simulink model "Couple_Tank"  (R2018b)
settings: Solver=ode5  StartTime=0.0  StopTime=1000  FixedStep=0.01  RelTol=1e-3  EnableMultiTasking=on
undefined symbols (not defined in the file or in its folder): sgn
settings Model: Creator=DUYLINH  LastModifiedBy=daiba
settings DataIOCC: LimitDataPoints=on  SaveFormat=Array
settings OptimizationCC: LifeSpan=inf
settings DebuggingCC: SFUnexpectedBacktrackingDiag=warning  SFNoUnconditionalDefaultTransitionDiag=warning  SFExecutionAtInitializationDiag=none
settings HardwareCC: ProdBitPerPointer=32  ProdBitPerSizeT=32  ProdBitPerPtrDiffT=32  ProdLargestAtomicFloat=None  ProdIntDivRoundTo=Undefined  ProdEndianess=Unspecified  ProdWordSize=32  ProdHWDeviceType=32-bit Generic
settings ModelReferenceCC: PropagateSignalLabelsOutOfModel=off
settings SFSimCC: SimUseLocalCustomCode=off
settings RTWCC: RTWUseLocalCustomCode=off
settings CodeAppCC: StateflowObjectComments=on
settings GRTTargetCC: TargetLangStandard=C89/C90 (ANSI)  GeneratePreprocessorConditionals=Disable all
settings ConfigComp: CovMetricSettings=dw  CovHtmlReporting=on  CovSaveCumulativeToWorkspaceVar=on  CovSaveSingleToWorkspaceVar=on  CovExternalEMLEnable=off

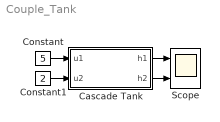
== system Couple_Tank ==
  " Cascade Tank" : Subsystem  mask{AA1=15, AA2=10, a1=0.3, a2=0.15, a12=0.1, k1=0.25, k2=0.2, Cd1=0.6, Cd2=0.6, Cd12=0.5, g=9.81, h1_zero=1, h2_zero=0.5}
      mask prompts: AA1 "Tiet dien ngang tank_1"; AA2 "Tiet dien ngang tank_2"; a1 "Tiet dien van xa tank_1"; a2 "Tiet dien van xa tank_2"; a12 "Tiet dien van xa giua 2 tank"; k1 "He so ti le cong suat may bom 1"; k2 "He so ti le cong suat may bom 2"; Cd1 "He so xa tank_1"; Cd2 "He so xa tank_2"; Cd12 "He so xa giua 2 tank"; g "Gia toc trong truong"; h1_zero "Muc nuoc tank_1 ban dau"; h2_zero "Muc nuoc tank_2 ban dau"
  Constant : Constant  Value=5
  Constant1 : Constant  Value=2
  Scope : Scope  NumInputPorts=2
  wires:
  " Cascade Tank"/1(h1) -> Scope/1
  Constant/1 -> " Cascade Tank"/1(u1)
  " Cascade Tank"/2(h2) -> Scope/2
  Constant1/1 -> " Cascade Tank"/2(u2)

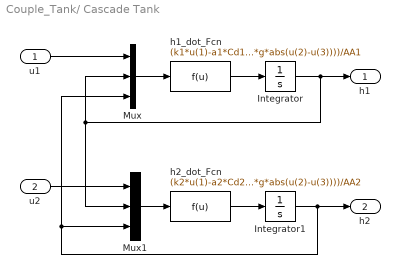
== system Couple_Tank/ Cascade Tank ==
  u1 : Inport
  u2 : Inport  Port=2
  Integrator : Integrator  InitialCondition=h1_zero
  Integrator1 : Integrator  InitialCondition=h2_zero
  Mux : Mux  Inputs=3
  Mux1 : Mux  Inputs=3
  h1_dot_Fcn : Fcn  Expr=(k1*u(1)-a1*Cd1*sqrt(2*g*u(2))-Cd12*sgn(u(2)-u(3))*a12*sqrt(2*g*abs(u(2)-u(3))))/AA1
  h2_dot_Fcn : Fcn  Expr=(k2*u(1)-a2*Cd2*sqrt(2*g*u(3))-Cd12*sgn(u(3)-u(2))*a12*sqrt(2*g*abs(u(2)-u(3))))/AA2
  h1 : Outport
  h2 : Outport  Port=2
  wires:
  Mux/1 -> h1_dot_Fcn/1
  h1_dot_Fcn/1 -> Integrator/1
  Integrator/1 -> Mux/2, Mux1/2, h1/1
  h2_dot_Fcn/1 -> Integrator1/1
  Mux1/1 -> h2_dot_Fcn/1
  Integrator1/1 -> Mux/3, Mux1/3, h2/1
  u1/1 -> Mux/1
  u2/1 -> Mux1/1
